simulink model "punto2"  (R2015a)
settings: Solver=ode45  StartTime=0.0  StopTime=10.0  RelTol=1e-3
libraries: cstblocks x1
settings Model: Creator=Jose Roldan  LastModifiedBy=Jose Roldan

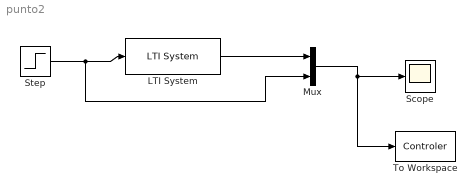
== system punto2 ==
  LTI System : cstblocks/LTI System  sys=G  IC=[]
  Mux : Mux  Inputs=2
  Scope : Scope
  Step : Step  SampleTime=0
  To Workspace : ToWorkspace  VariableName=Controler  SaveFormat=Timeseries  SampleTime=-1
  wires:
  Step/1 -> Mux/2, LTI System/1
  LTI System/1 -> Mux/1
  Mux/1 -> To Workspace/1, Scope/1
